simulink model "TL_model"  (R2015b)
settings: Solver=VariableStepAuto  StartTime=0.0  StopTime=50  RelTol=1e-3
settings Model: Creator=loicgelle  LastModifiedBy=loicgelle

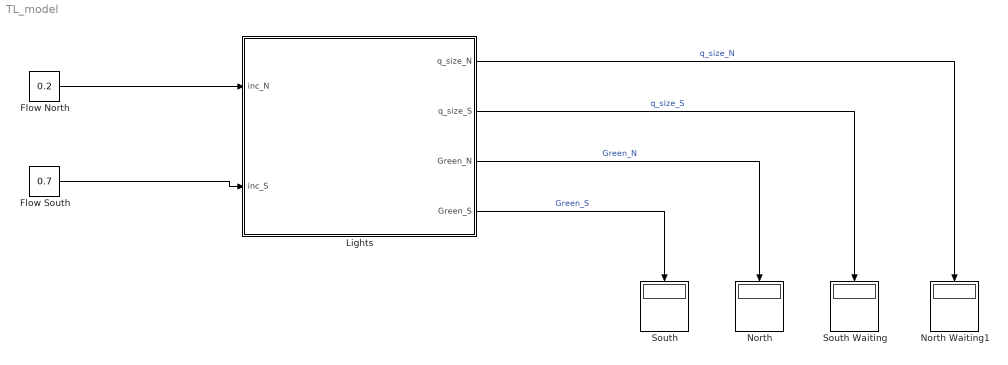
== system TL_model ==
  " North" : Display
  " North Waiting1" : Display
  " South" : Display
  " South Waiting" : Display
  Flow North : Constant  Value=0.2
  Flow South : Constant  Value=0.7
  Lights : Stateflow chart  TreatAsAtomicUnit=on  VariantControl=Variant1
  wires:
  Lights/3(Green_N) -> " North"/1  "Green_N"
  Lights/4(Green_S) -> " South"/1  "Green_S"
  Flow North/1 -> Lights/1(inc_N)
  Flow South/1 -> Lights/2(inc_S)
  Lights/2(q_size_S) -> " South Waiting"/1  "q_size_S"
  Lights/1(q_size_N) -> " North Waiting1"/1  "q_size_N"

== stateflow chart TL_model/Lights ==
  settings: updateMethod=CONTINUOUS
  state LightsController [parallel]
    settings: executionOrder=1
    state GreenS
      entry:
      t = 0;
      Green_S = 1;
      during:
      t_dot = 1;
      exit:
      Green_S = 0;
    state GreenN
      entry:
      t = 0;
      Green_N = 1;
      during:
      t_dot = 1;
      exit:
      Green_N = 0;
    state Clear
      entry:
      Green_N = 0;
      Green_S = 0;
    GreenN -> GreenS [order 1] : [q_size_N <= 0]
    GreenN -> GreenS [order 2] : [t >= t_N]
    Clear -> GreenN [order 2] : after(1, sec)
        | [q_size_N + q_size_S > 0]
        | {computeTimes()}
    GreenS -> Clear [order 2] : [q_size_S <= 0]
    GreenS -> Clear [order 1] : [t >= t_S]
    Clear -> Clear [order 1] : after(1, sec)
        | [q_size_N + q_size_S <= 0]
    (default) -> Clear
  state Queue_Handler_N [parallel]
    settings: executionOrder=2
    state Red
      during:
      q_size_N_dot = inc_N;
    state Green
      during:
      q_size_N_dot = inc_N - out;
    Queue_Handler_N.Green -> Queue_Handler_N.Red : [Green_N == 0]
    Queue_Handler_N.Red -> Queue_Handler_N.Green : [Green_N == 1]
    (default) -> Queue_Handler_N.Red
  state Queue_Handler_S [parallel]
    settings: executionOrder=3
    state Red
      during:
      q_size_S_dot = inc_S;
    state Green
      during:
      q_size_S_dot = inc_S - out;
    Queue_Handler_S.Green -> Queue_Handler_S.Red : [Green_S == 0]
    Queue_Handler_S.Red -> Queue_Handler_S.Green : [Green_S == 1]
    (default) -> Queue_Handler_S.Red
  data: q_size_N output =0; q_size_S output =0; t_N local =0; t_S local =0; cycle_duration constant double =10; Green_N output; Green_S output; data local; inc_N input; inc_S input; out constant double =2; t local =0
  data q_size_N settings: updateMethod=SF_CONTINUOUS_TIME_DATA
  data q_size_S settings: updateMethod=SF_CONTINUOUS_TIME_DATA
  data t settings: updateMethod=SF_CONTINUOUS_TIME_DATA
  function computeTimes:
    | function computeTimes
    |  
    | t_N = cycle_duration / 2;
    | t_S = cycle_duration / 2;
